simulink model "Indices_Error_PModeloE_Sintonizaciones"  (R2019b)
settings: Solver=VariableStepAuto  StartTime=0.0  StopTime=10.1  RelTol=1e-3  EnableMultiTasking=on
libraries: simulink x4
settings Model: Creator=alber  LastModifiedBy=belindabrown
settings DataIOCC: ReturnWorkspaceOutputs=off
settings OptimizationCC: LifeSpan=inf
settings DebuggingCC: SFUnexpectedBacktrackingDiag=warning  SFNoUnconditionalDefaultTransitionDiag=warning  ArithmeticOperatorsInVariantConditions=warning
settings SFSimCC: SimUseLocalCustomCode=off  CustomCodeUndefinedFunction=UseInterfaceOnly
settings RTWCC: RTWUseLocalCustomCode=off
settings CodeAppCC: StateflowObjectComments=on
settings GRTTargetCC: TargetLangStandard=C89/C90 (ANSI)  GeneratePreprocessorConditionals=Disable all
settings ConfigComp: CovMetricSettings=dw  CovHtmlReporting=on  CovSaveCumulativeToWorkspaceVar=on  CovSaveSingleToWorkspaceVar=on  CovExternalEMLEnable=off

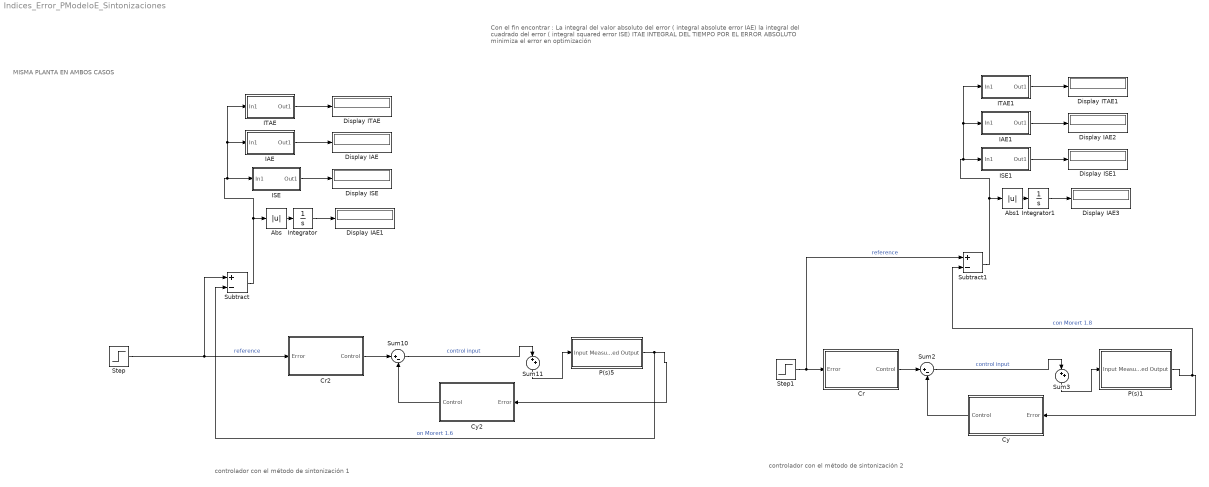
== system Indices_Error_PModeloE_Sintonizaciones ==
  note: MISMA PLANTA EN AMBOS CASOS
  note: controlador con el método de sintonización 2
  note: Con el fin encontrar :
      |
      | La integral del valor absoluto del error
      | ( integral absolute error IAE)
      |
      | la integral del cuadrado del error ( integral squared error ISE)
      |
      | ITAE INTEGRAL DEL TIEMPO POR EL ERROR ABSOLUTO minimiza el error en optimización
  note: controlador con el método de sintonización 1
  Abs : Abs
  Abs1 : Abs
  Cr : Subsystem
  Cr2 : Subsystem
  Cy : Subsystem
  Cy2 : Subsystem
  Display IAE{,1..3} (4 alike) : Display
  Display ISE : Display
  Display ISE1 : Display
  Display ITAE : Display
  Display ITAE1 : Display
  IAE : Subsystem
      mask help:
      | IAE performacne index
      |
      | output = int |input| dt
      mask Display:
      | disp('IAE')
      | port_label('input',1,'e')
      | port_label('output',1,'iae')
  IAE1 : Subsystem
      mask help:
      | IAE performacne index
      |
      | output = int |input| dt
      mask Display:
      | disp('IAE')
      | port_label('input',1,'e')
      | port_label('output',1,'iae')
  ISE : Subsystem
      mask help:
      | ISE performance index
      |
      | output = int (input)^2 dt
      mask Display:
      | disp('ISE')
      | port_label('input',1,'e')
      | port_label('output',1,'ise')
  ISE1 : Subsystem
      mask help:
      | ISE performance index
      |
      | output = int (input)^2 dt
      mask Display:
      | disp('ISE')
      | port_label('input',1,'e')
      | port_label('output',1,'ise')
  ITAE : Subsystem
      mask help:
      | ITAE performance index
      |
      | output = int t|input| dt
      mask Display:
      | disp('ITAE')
      | port_label('input',1,'e')
      | port_label('output',1,'itae')
  ITAE1 : Subsystem
      mask help:
      | ITAE performance index
      |
      | output = int t|input| dt
      mask Display:
      | disp('ITAE')
      | port_label('input',1,'e')
      | port_label('output',1,'itae')
  Integrator : Integrator
  Integrator1 : Integrator
  P(s)1 : Subsystem
  P(s)5 : Subsystem
  Step : Step  Time=10  SampleTime=0
  Step1 : Step  Time=10  SampleTime=0
  Subtract : Sum  Inputs=+-
  Subtract1 : Sum  Inputs=+-
  Sum10 : Sum  Inputs=|+-
  Sum11 : Sum  Inputs=|++
  Sum2 : Sum  Inputs=|+-
  Sum3 : Sum  Inputs=|++
  wires:
  IAE/1(Out1) -> Display IAE/1
  ISE/1(Out1) -> Display ISE/1
  ITAE/1(Out1) -> Display ITAE/1
  Abs/1 -> Integrator/1
  Integrator/1 -> Display IAE1/1
  P(s)5/1(Measured Output) -> Subtract/2, Cy2/1(Error)  "on Morert 1.6"
  Sum10/1 -> Sum11/1  "control input"
  Sum11/1 -> P(s)5/1(Input)
  Cr2/1(Control) -> Sum10/1
  Cy2/1(Control) -> Sum10/2
  Step/1 -> Subtract/1, Cr2/1(Error)  "reference"
  Subtract/1 -> ITAE/1(In1), IAE/1(In1), ISE/1(In1), Abs/1
  P(s)1/1(Measured Output) -> Subtract1/2, Cy/1(Error)  "con Morert 1.8"
  Sum2/1 -> Sum3/1  "control input"
  Sum3/1 -> P(s)1/1(Input)
  Cr/1(Control) -> Sum2/1
  Cy/1(Control) -> Sum2/2
  Step1/1 -> Subtract1/1, Cr/1(Error)  "reference"
  IAE1/1(Out1) -> Display IAE2/1
  ISE1/1(Out1) -> Display ISE1/1
  ITAE1/1(Out1) -> Display ITAE1/1
  Abs1/1 -> Integrator1/1
  Integrator1/1 -> Display IAE3/1
  Subtract1/1 -> ITAE1/1(In1), IAE1/1(In1), ISE1/1(In1), Abs1/1

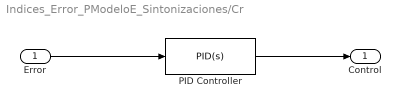
== system Indices_Error_PModeloE_Sintonizaciones/Cr ==
  Error : Inport
  PID Controller : simulink/Continuous/PID Controller  Controller=PID  Form=Ideal  TimeDomain=Continuous-time  SampleTime=-1  IntegratorMethod=Forward Euler  FilterMethod=Forward Euler  ControllerParametersSource=internal  P=1.57  I=1/9.59  D=0.011  UseFilter=on  N=1000  TunerSelectOption=Transfer Function Based (PID Tuner App)  InitialConditionSource=internal  InitialConditionForIntegrator=0  InitialConditionForFilter=0  DifferentiatorICPrevScaledInput=0  ExternalReset=none  TrackingMode=off  Kt=1  LimitOutput=off  UpperSaturationLimit=inf  LowerSaturationLimit=-inf  LinearizeAsGain=on  AntiWindupMode=none  Kb=1  POutMin=[]  POutMax=[]  IOutMin=[]  IOutMax=[]  DOutMin=[]  DOutMax=[]  NOutMin=[]  NOutMax=[]  SumOutMin=[]  SumOutMax=[]  SaturationOutMin=[]  SaturationOutMax=[]  PParamMin=[]  PParamMax=[]  IParamMin=[]  IParamMax=[]  DParamMin=[]  DParamMax=[]  NParamMin=[]  NParamMax=[]  KbParamMin=[]  KbParamMax=[]  KtParamMin=[]  KtParamMax=[]  KbOutMin=[]  KbOutMax=[]  KtOutMin=[]  KtOutMax=[]  IntegratorOutMin=[]  IntegratorOutMax=[]  FilterOutMin=[]  FilterOutMax=[]  SumI1OutMin=[]  SumI1OutMax=[]  SumI2OutMin=[]  SumI2OutMax=[]  SumI3OutMin=[]  SumI3OutMax=[]  SumI4OutMin=[]  SumI4OutMax=[]  SumDOutMin=[]  SumDOutMax=[]  DifferentiatorOutMin=[]  DifferentiatorOutMax=[]  FilterDiffOutCoefMin=[]  FilterDiffOutCoefMax=[]  ReciprocalOutMin=[]  ReciprocalOutMax=[]  SumDenOutMin=[]  SumDenOutMax=[]  SumNumOutMin=[]  SumNumOutMax=[]  DivideOutMin=[]  DivideOutMax=[]  IntegratorContinuousStateAttributes=''  IntegratorStateMustResolveToSignalObject=off  IntegratorRTWStateStorageClass=Auto  FilterContinuousStateAttributes=''  FilterStateMustResolveToSignalObject=off  FilterRTWStateStorageClass=Auto  ParallelPVariant=Passthrough  IdealPVariant=InternalParameters  IVariant=InternalParameters  DVariant=InternalParameters  IntegratorVariant=Continuous  SatVariant=Disabled  AWVariant=Passthrough  PCopyVariant=Disabled  TRVariant=Disabled  FdbkBlocksVariant=Forward  IdealPFdbkVariant=Disabled  SatFdbkVariant=Disabled  DerivativeFilterVariant=ContFilter  NVariant=InternalParameters  NCopyVariant=Disabled  FilterICVariant=InternalICsFilter  IntegratorICVariant=InternalICs  ExternalResetVariant=Disabled  TRSumVariant=Passthrough  SumFdbkVariant=Disabled  SumVariant=Sum_PID
  Control : Outport
  wires:
  PID Controller/1 -> Control/1
  Error/1 -> PID Controller/1

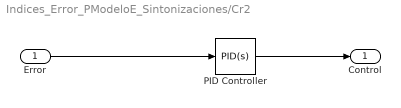
== system Indices_Error_PModeloE_Sintonizaciones/Cr2 ==
  Error : Inport
  PID Controller : simulink/Continuous/PID Controller  Controller=PID  Form=Ideal  TimeDomain=Continuous-time  SampleTime=-1  IntegratorMethod=Forward Euler  FilterMethod=Forward Euler  ControllerParametersSource=internal  P=1.82  I=1/12.82  D=0.0092  UseFilter=on  N=1000  TunerSelectOption=Transfer Function Based (PID Tuner App)  InitialConditionSource=internal  InitialConditionForIntegrator=0  InitialConditionForFilter=0  DifferentiatorICPrevScaledInput=0  ExternalReset=none  TrackingMode=off  Kt=1  LimitOutput=off  UpperSaturationLimit=inf  LowerSaturationLimit=-inf  LinearizeAsGain=on  AntiWindupMode=none  Kb=1  POutMin=[]  POutMax=[]  IOutMin=[]  IOutMax=[]  DOutMin=[]  DOutMax=[]  NOutMin=[]  NOutMax=[]  SumOutMin=[]  SumOutMax=[]  SaturationOutMin=[]  SaturationOutMax=[]  PParamMin=[]  PParamMax=[]  IParamMin=[]  IParamMax=[]  DParamMin=[]  DParamMax=[]  NParamMin=[]  NParamMax=[]  KbParamMin=[]  KbParamMax=[]  KtParamMin=[]  KtParamMax=[]  KbOutMin=[]  KbOutMax=[]  KtOutMin=[]  KtOutMax=[]  IntegratorOutMin=[]  IntegratorOutMax=[]  FilterOutMin=[]  FilterOutMax=[]  SumI1OutMin=[]  SumI1OutMax=[]  SumI2OutMin=[]  SumI2OutMax=[]  SumI3OutMin=[]  SumI3OutMax=[]  SumI4OutMin=[]  SumI4OutMax=[]  SumDOutMin=[]  SumDOutMax=[]  DifferentiatorOutMin=[]  DifferentiatorOutMax=[]  FilterDiffOutCoefMin=[]  FilterDiffOutCoefMax=[]  ReciprocalOutMin=[]  ReciprocalOutMax=[]  SumDenOutMin=[]  SumDenOutMax=[]  SumNumOutMin=[]  SumNumOutMax=[]  DivideOutMin=[]  DivideOutMax=[]  IntegratorContinuousStateAttributes=''  IntegratorStateMustResolveToSignalObject=off  IntegratorRTWStateStorageClass=Auto  FilterContinuousStateAttributes=''  FilterStateMustResolveToSignalObject=off  FilterRTWStateStorageClass=Auto  ParallelPVariant=Passthrough  IdealPVariant=InternalParameters  IVariant=InternalParameters  DVariant=InternalParameters  IntegratorVariant=Continuous  SatVariant=Disabled  AWVariant=Passthrough  PCopyVariant=Disabled  TRVariant=Disabled  FdbkBlocksVariant=Forward  IdealPFdbkVariant=Disabled  SatFdbkVariant=Disabled  DerivativeFilterVariant=ContFilter  NVariant=InternalParameters  NCopyVariant=Disabled  FilterICVariant=InternalICsFilter  IntegratorICVariant=InternalICs  ExternalResetVariant=Disabled  TRSumVariant=Passthrough  SumFdbkVariant=Disabled  SumVariant=Sum_PID
  Control : Outport
  wires:
  PID Controller/1 -> Control/1
  Error/1 -> PID Controller/1

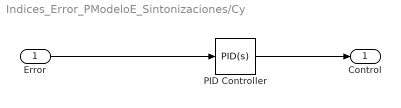
== system Indices_Error_PModeloE_Sintonizaciones/Cy ==
  Error : Inport
  PID Controller : simulink/Continuous/PID Controller  Controller=PID  Form=Ideal  TimeDomain=Continuous-time  SampleTime=-1  IntegratorMethod=Forward Euler  FilterMethod=Forward Euler  ControllerParametersSource=internal  P=1.57  I=1/9.59  D=0.011  UseFilter=on  N=1000  TunerSelectOption=Transfer Function Based (PID Tuner App)  InitialConditionSource=internal  InitialConditionForIntegrator=0  InitialConditionForFilter=0  DifferentiatorICPrevScaledInput=0  ExternalReset=none  TrackingMode=off  Kt=1  LimitOutput=off  UpperSaturationLimit=inf  LowerSaturationLimit=-inf  LinearizeAsGain=on  AntiWindupMode=none  Kb=1  POutMin=[]  POutMax=[]  IOutMin=[]  IOutMax=[]  DOutMin=[]  DOutMax=[]  NOutMin=[]  NOutMax=[]  SumOutMin=[]  SumOutMax=[]  SaturationOutMin=[]  SaturationOutMax=[]  PParamMin=[]  PParamMax=[]  IParamMin=[]  IParamMax=[]  DParamMin=[]  DParamMax=[]  NParamMin=[]  NParamMax=[]  KbParamMin=[]  KbParamMax=[]  KtParamMin=[]  KtParamMax=[]  KbOutMin=[]  KbOutMax=[]  KtOutMin=[]  KtOutMax=[]  IntegratorOutMin=[]  IntegratorOutMax=[]  FilterOutMin=[]  FilterOutMax=[]  SumI1OutMin=[]  SumI1OutMax=[]  SumI2OutMin=[]  SumI2OutMax=[]  SumI3OutMin=[]  SumI3OutMax=[]  SumI4OutMin=[]  SumI4OutMax=[]  SumDOutMin=[]  SumDOutMax=[]  DifferentiatorOutMin=[]  DifferentiatorOutMax=[]  FilterDiffOutCoefMin=[]  FilterDiffOutCoefMax=[]  ReciprocalOutMin=[]  ReciprocalOutMax=[]  SumDenOutMin=[]  SumDenOutMax=[]  SumNumOutMin=[]  SumNumOutMax=[]  DivideOutMin=[]  DivideOutMax=[]  IntegratorContinuousStateAttributes=''  IntegratorStateMustResolveToSignalObject=off  IntegratorRTWStateStorageClass=Auto  FilterContinuousStateAttributes=''  FilterStateMustResolveToSignalObject=off  FilterRTWStateStorageClass=Auto  ParallelPVariant=Passthrough  IdealPVariant=InternalParameters  IVariant=InternalParameters  DVariant=InternalParameters  IntegratorVariant=Continuous  SatVariant=Disabled  AWVariant=Passthrough  PCopyVariant=Disabled  TRVariant=Disabled  FdbkBlocksVariant=Forward  IdealPFdbkVariant=Disabled  SatFdbkVariant=Disabled  DerivativeFilterVariant=ContFilter  NVariant=InternalParameters  NCopyVariant=Disabled  FilterICVariant=InternalICsFilter  IntegratorICVariant=InternalICs  ExternalResetVariant=Disabled  TRSumVariant=Passthrough  SumFdbkVariant=Disabled  SumVariant=Sum_PID
  Control : Outport
  wires:
  PID Controller/1 -> Control/1
  Error/1 -> PID Controller/1

== system Indices_Error_PModeloE_Sintonizaciones/Cy2 ==
  Error : Inport
  PID Controller : simulink/Continuous/PID Controller  Controller=PID  Form=Ideal  TimeDomain=Continuous-time  SampleTime=-1  IntegratorMethod=Forward Euler  FilterMethod=Forward Euler  ControllerParametersSource=internal  P=1.82  I=1/12.82  D=0.0092  UseFilter=on  N=1000  TunerSelectOption=Transfer Function Based (PID Tuner App)  InitialConditionSource=internal  InitialConditionForIntegrator=0  InitialConditionForFilter=0  DifferentiatorICPrevScaledInput=0  ExternalReset=none  TrackingMode=off  Kt=1  LimitOutput=off  UpperSaturationLimit=inf  LowerSaturationLimit=-inf  LinearizeAsGain=on  AntiWindupMode=none  Kb=1  POutMin=[]  POutMax=[]  IOutMin=[]  IOutMax=[]  DOutMin=[]  DOutMax=[]  NOutMin=[]  NOutMax=[]  SumOutMin=[]  SumOutMax=[]  SaturationOutMin=[]  SaturationOutMax=[]  PParamMin=[]  PParamMax=[]  IParamMin=[]  IParamMax=[]  DParamMin=[]  DParamMax=[]  NParamMin=[]  NParamMax=[]  KbParamMin=[]  KbParamMax=[]  KtParamMin=[]  KtParamMax=[]  KbOutMin=[]  KbOutMax=[]  KtOutMin=[]  KtOutMax=[]  IntegratorOutMin=[]  IntegratorOutMax=[]  FilterOutMin=[]  FilterOutMax=[]  SumI1OutMin=[]  SumI1OutMax=[]  SumI2OutMin=[]  SumI2OutMax=[]  SumI3OutMin=[]  SumI3OutMax=[]  SumI4OutMin=[]  SumI4OutMax=[]  SumDOutMin=[]  SumDOutMax=[]  DifferentiatorOutMin=[]  DifferentiatorOutMax=[]  FilterDiffOutCoefMin=[]  FilterDiffOutCoefMax=[]  ReciprocalOutMin=[]  ReciprocalOutMax=[]  SumDenOutMin=[]  SumDenOutMax=[]  SumNumOutMin=[]  SumNumOutMax=[]  DivideOutMin=[]  DivideOutMax=[]  IntegratorContinuousStateAttributes=''  IntegratorStateMustResolveToSignalObject=off  IntegratorRTWStateStorageClass=Auto  FilterContinuousStateAttributes=''  FilterStateMustResolveToSignalObject=off  FilterRTWStateStorageClass=Auto  ParallelPVariant=Passthrough  IdealPVariant=InternalParameters  IVariant=InternalParameters  DVariant=InternalParameters  IntegratorVariant=Continuous  SatVariant=Disabled  AWVariant=Passthrough  PCopyVariant=Disabled  TRVariant=Disabled  FdbkBlocksVariant=Forward  IdealPFdbkVariant=Disabled  SatFdbkVariant=Disabled  DerivativeFilterVariant=ContFilter  NVariant=InternalParameters  NCopyVariant=Disabled  FilterICVariant=InternalICsFilter  IntegratorICVariant=InternalICs  ExternalResetVariant=Disabled  TRSumVariant=Passthrough  SumFdbkVariant=Disabled  SumVariant=Sum_PID
  Control : Outport
  wires:
  PID Controller/1 -> Control/1
  Error/1 -> PID Controller/1

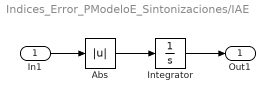
== system Indices_Error_PModeloE_Sintonizaciones/IAE ==
  In1 : Inport
  Abs : Abs
  Integrator : Integrator
  Out1 : Outport
  wires:
  In1/1 -> Abs/1
  Integrator/1 -> Out1/1
  Abs/1 -> Integrator/1

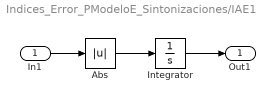
== system Indices_Error_PModeloE_Sintonizaciones/IAE1 ==
  In1 : Inport
  Abs : Abs
  Integrator : Integrator
  Out1 : Outport
  wires:
  In1/1 -> Abs/1
  Integrator/1 -> Out1/1
  Abs/1 -> Integrator/1

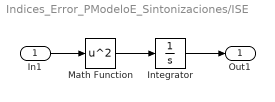
== system Indices_Error_PModeloE_Sintonizaciones/ISE ==
  In1 : Inport
  Integrator : Integrator
  Math Function : Math  Operator=square  SaturateOnIntegerOverflow=on
  Out1 : Outport
  wires:
  Math Function/1 -> Integrator/1
  Integrator/1 -> Out1/1
  In1/1 -> Math Function/1

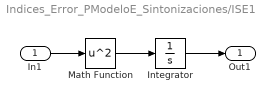
== system Indices_Error_PModeloE_Sintonizaciones/ISE1 ==
  In1 : Inport
  Integrator : Integrator
  Math Function : Math  Operator=square  SaturateOnIntegerOverflow=on
  Out1 : Outport
  wires:
  Math Function/1 -> Integrator/1
  Integrator/1 -> Out1/1
  In1/1 -> Math Function/1

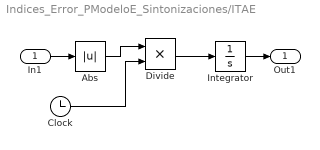
== system Indices_Error_PModeloE_Sintonizaciones/ITAE ==
  In1 : Inport
  Abs : Abs
  Clock : Clock
  Divide : Product  Inputs=**
  Integrator : Integrator
  Out1 : Outport
  wires:
  Integrator/1 -> Out1/1
  In1/1 -> Abs/1
  Divide/1 -> Integrator/1
  Abs/1 -> Divide/1
  Clock/1 -> Divide/2

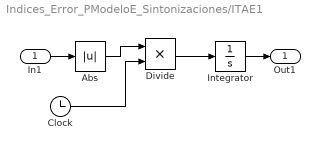
== system Indices_Error_PModeloE_Sintonizaciones/ITAE1 ==
  In1 : Inport
  Abs : Abs
  Clock : Clock
  Divide : Product  Inputs=**
  Integrator : Integrator
  Out1 : Outport
  wires:
  Integrator/1 -> Out1/1
  In1/1 -> Abs/1
  Divide/1 -> Integrator/1
  Abs/1 -> Divide/1
  Clock/1 -> Divide/2

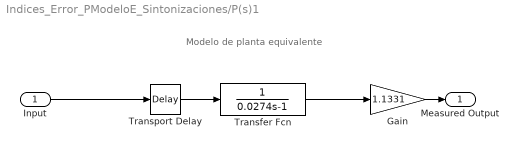
== system Indices_Error_PModeloE_Sintonizaciones/P(s)1 ==
  note: Modelo de planta equivalente
  Input : Inport
  Gain : Gain  Gain=1.1331
  Transfer Fcn : TransferFcn  Denominator=[0.0274 -1]
  Transport Delay : TransportDelay  DelayTime=0.020
  Measured Output : Outport
  wires:
  Input/1 -> Transport Delay/1
  Transport Delay/1 -> Transfer Fcn/1
  Gain/1 -> Measured Output/1
  Transfer Fcn/1 -> Gain/1

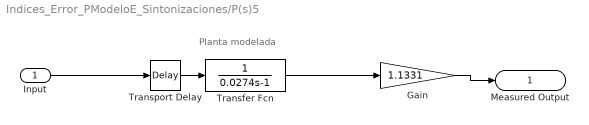
== system Indices_Error_PModeloE_Sintonizaciones/P(s)5 ==
  note: Planta modelada
  Input : Inport
  Gain : Gain  Gain=1.1331
  Transfer Fcn : TransferFcn  Denominator=[0.0274 -1]
  Transport Delay : TransportDelay  DelayTime=0.020
  Measured Output : Outport
  wires:
  Input/1 -> Transport Delay/1
  Transport Delay/1 -> Transfer Fcn/1
  Gain/1 -> Measured Output/1
  Transfer Fcn/1 -> Gain/1
